simulink model "HQEV_MiL_20160830_integrate"  (Simulink 8.3)
settings: Solver=FixedStepDiscrete  StartTime=0.0  StopTime=inf  FixedStep=0.01  RelTol=1e-3
PostLoadFcn:
  | , if any(exist('dsrtsu_mdlpostloadfcn', 'file') == [2, 3, 6]), try dsrtsu_mdlpostloadfcn('Execute', bdroot); catch fprintf('Error in PostLoadFcn (dsrtsu_mdlpostloadfcn) for model "%s":\n %s\n', bdroot, lasterr); end, end,
values from neighbouring files (symbols this model uses):
  Bat_C_Ah = 36    [parameter_V1.mat]
  Bat_ocv_xIndex = [5 10 20 30 40 50 60 70 80 90 95]    [parameter_V1.mat]
  Bat_ocv_z = [329 332 340 345 347 351 358 372 377 386 391]    [parameter_V1.mat]
  Bat_R_ohm_z = [4.41 3.46 1.57 1.07 0.76 0.63 0.55 0.44 0.41 0.4 0.4 3.14 ... (66 elements, 11x6)]    [parameter_V1.mat]
  Bat_SOC_Init = 90    [parameter_V1.mat]
  Env_hum_pct_Ambient = 30    [parameter_V1.mat]
  Env_Slope_deg = 0    [parameter_V1.mat]
  Env_Temp_degC_Ambient = 25    [parameter_V1.mat]
  Env_v_kmph_HWind = 0    [parameter_V1.mat]
  Reducer_F_i = 7.23    [parameter_V1.mat]
  Reducer_R_i = 7.23    [parameter_V1.mat]
  Veh =     [parameter_V1.mat]
  Veh_A_m2_Fr = 2.246    [parameter_V1.mat]
  Veh_F_Brake =     [parameter_V1.mat]
  Veh_fac_AirDrag = 0.326    [parameter_V1.mat]
  Veh_fac_WhDragFrict_0 = 0.011    [parameter_V1.mat]
  Veh_g_mps2_C = 9.81    [parameter_V1.mat]
  Veh_GainBrake =     [parameter_V1.mat]
  Veh_h_m_COGHigh = 0.5    [parameter_V1.mat]
  Veh_J_kgm2_Wh = 1.3635    [parameter_V1.mat]
  Veh_L_m_AxlBas = 2.63    [parameter_V1.mat]
  Veh_M_kg = 1427    [parameter_V1.mat]
  Veh_mu_Brake = 0.4    [parameter_V1.mat]
  Veh_mu_Tyre =     [parameter_V1.mat]
  Veh_num_FrictPair = 8    [parameter_V1.mat]
  Veh_pct_Brk = 70    [parameter_V1.mat]
  Veh_r_dyn =     [parameter_V1.mat]
  Veh_r_m_BrkDisk = 0.136    [parameter_V1.mat]
  Veh_rho_kgpm3_Air = 1.2258    [parameter_V1.mat]
undefined symbols (not defined in the file or in its folder): DiscIntNeverNeededParam, p_bool_False_M, p_bool_True_M
libraries: BaseOperationLib_Browser x38, simulink x9, DTQC_lib x1, ERR_lib x1, MQM_lib x1, PTCL_lib x1, PUD_lib x1, TQD_lib x1, TQR_lib x1, VMM_lib x1, ACCA_lib x1, BBCA_lib x1
(part 1 of 15)
settings Model: DSRTSU_INTERNAL_RTI_VER=380  DSRTSU_INTERNAL_RTI_TYPE=rti1401  RTICANMMDATA=struct('GeneralSetupData',struct('modelroot','G:\2015\A0EV\MIL_Model_1118\200_Model\230_Integration','generalsettings',struct('filesettings',struct('destfolder',struct('Name','RTICANMM_FILES','Check',1),'buildfolder',struct('Name','.','Check',1),'AbsDestfolder',struct('Name','G:\2015\A0EV\MIL_Model_1118\200_Model\230_Integration\RTICANMM_FILES'),'AbsBuildfolder',struct('Name','G:\2015\A0EV\MIL_Model_1118\200_Model\230_Integration'))),'options',struct('addpaths',1,'rmpaths',1,'addtrcexclusion',logical(1),'cannavigator',struct('checkmonitoring',0,'serviceno','31','hostservicedefheader',struct('name','x','path','x')),'show_usrtrc',0,'use_usrtrc',0),'advanced',struct('options',[1 1 1 1 1 1 1 1 1 1 1 1 1 1 1 1 1 1 1 1 1 1 1 1 1 1 1 1 1 1 1 1 1 1 1 1 1 1 1 1 1 1 1 1 1 1 1 1 1 1 1 1 1 1 1 1 1 1 1 1 1 1 1 1 1 1 1 1 1 1 1 1 1 1 1 1 1 1 1 1 1 1 1 1 1 1 1 1 1 1 1 1 1 1 1 1 1 1 1 1]),'MPSetup',{{}},'modelname','A0EV_HuanJing_1214','block','A0EV_HuanJing_1214'))  Creator=wuaibin  LastModifiedBy=yangfuchun
settings DataIOCC: SaveFormat=StructureWithTime
settings OptimizationCC: BlockReduction=off  ExpressionDepthLimit=2147483647
settings DebuggingCC: FcnCallInpInsideContextMsg=UseLocalSettings
settings HardwareCC: ProdIntDivRoundTo=Zero  ProdEndianess=BigEndian  ProdHWDeviceType=Generic->Custom  TargetIntDivRoundTo=Zero  TargetEndianess=BigEndian  TargetHWDeviceType=Generic->Custom
settings RTWCC: GenerateMakefile=off  TemplateMakefile=grt_msvc.tmf  Description="Visual C/C++ Project Makefile only for the \"grt\" target"  ProcessScript=grt_make_rtw_hook

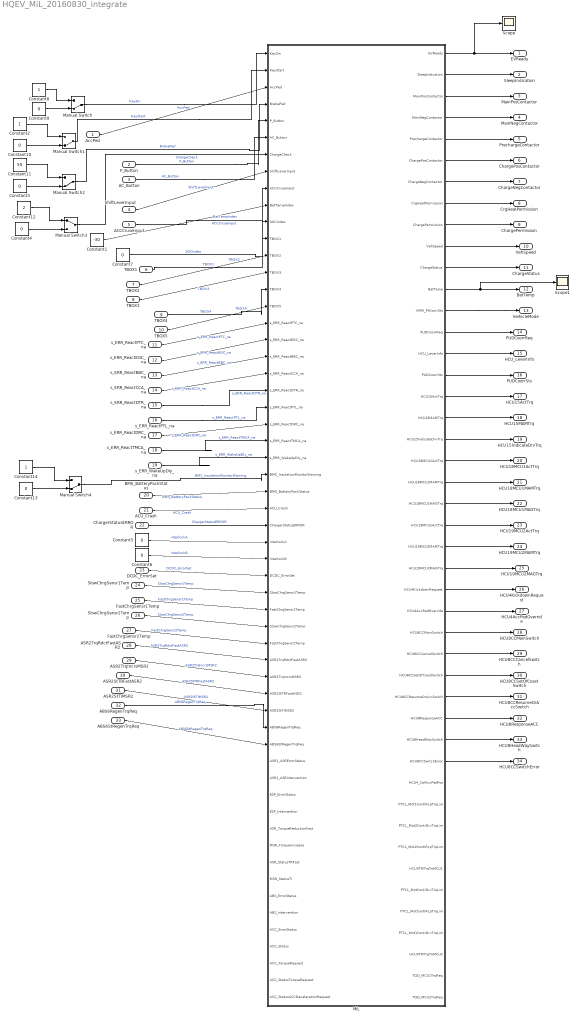
== system HQEV_MiL_20160830_integrate ==
  AccPed : Inport
  P_Button : Inport  Port=2
  AC_Button : Inport  Port=3
  ShiftLeverInput : Inport  Port=4
  ACCCruseInput : Inport  Port=5
  TBOX1 : Inport  Port=6
  TBOX2 : Inport  Port=7
  TBOX3 : Inport  Port=8
  TBOX4 : Inport  Port=9
  TBOX5 : Inport  Port=10
  s_ERR_ReactPTC_na : Inport  Port=11
  s_ERR_ReactEGC_na : Inport  Port=12
  s_ERR_ReactBBC_na : Inport  Port=13
  s_ERR_ReactCCA_na : Inport  Port=14
  s_ERR_ReactDTR_na : Inport  Port=15
  s_ERR_ReactPTL_na : Inport  Port=16
  s_ERR_ReactDRC_na : Inport  Port=17
  s_ERR_ReactTMCA_na : Inport  Port=18
  s_ERR_WakeUpDly_na : Inport  Port=19
  BMS_BatteryPackStatus : Inport  Port=20
  ACU_Crash : Inport  Port=21
  ChargerStatusERROR : Inport  Port=22
  DCDC_ErrorSet : Inport  Port=23
  SlowChrgSensr1Temp : Inport  Port=24
  FastChrgSensr1Temp : Inport  Port=25
  SlowChrgSensr2Temp : Inport  Port=26
  FastChrgSensr2Temp : Inport  Port=27
  ASR2TrqRdctFastASR2 : Inport  Port=28
  ASR2TrqIncrsMSR2 : Inport  Port=29
  ASR2StTRFastASR2 : Inport  Port=30
  ASR2StTIMSR2 : Inport  Port=31
  ABS6RegenTrqReq : Inport  Port=32
  ABS6StRegenTrqReq : Inport  Port=33
  Constant1 : Constant  Value=-30
  Constant{3..7,9..10,13} (8 alike) : Constant  Value=0
  Constant11 : Constant  Value=50
  Constant12 : Constant  Value=2
  Constant14 : Constant
  Constant2 : Constant
  Constant8 : Constant
  Manual Switch{,1..2,4} (4 alike) : ManualSwitch  CurrentSetting=0
  Manual Switch3 : ManualSwitch
  MiL : Subsystem
  Scope : Scope
      settings: YMin=1.9  YMax=2.1
  Scope1 : Scope
      settings: YMin=1.9  YMax=2.1
  EVReady : Outport
  SleepIndication : Outport  Port=2
  MainPosContactor : Outport  Port=3
  MainNegContactor : Outport  Port=4
  PrechargeContactor : Outport  Port=5
  ChargePosContactor : Outport  Port=6
  ChargeNegContactor : Outport  Port=7
  CrgHeatPermission : Outport  Port=8
  ChargePermission : Outport  Port=9
  VehSpeed : Outport  Port=10
  ChargeStatus : Outport  Port=11
  BatTemp : Outport  Port=12
  VeihicleMode : Outport  Port=13
  PUDCoorrReq : Outport  Port=14
  HCU_LeverInfo : Outport  Port=15
  PUDCoorrSts : Outport  Port=16
  HCU15ActTrq : Outport  Port=17
  HCU15MAMTrq : Outport  Port=18
  HCU15IndicateDrvTrq : Outport  Port=19
  HCU18MCU1ActTrq : Outport  Port=20
  HCU18MCU1MAMTrq : Outport  Port=21
  HCU18MCU1MAGTrq : Outport  Port=22
  HCU19MCU2ActTrq : Outport  Port=23
  HCU19MCU2MAMTrq : Outport  Port=24
  HCU19MCU2MAGTrq : Outport  Port=25
  HCU4KickdownRequest : Outport  Port=26
  HCU4AccPedOverride : Outport  Port=27
  HCU8CCMainSwitch : Outport  Port=28
  HCU8CCCancelSwitch : Outport  Port=29
  HCU8CCSetOfCoastSwitch : Outport  Port=30
  HCU8CCResumeOrAccSwitch : Outport  Port=31
  HCU8ResponseACC : Outport  Port=32
  HCU8HeadWaySwitch : Outport  Port=33
  HCU8CCSwitchError : Outport  Port=34
  wires:
  MiL/9(ChargePermission) -> ChargePermission/1
  MiL/4(MainNegContactor) -> MainNegContactor/1
  MiL/1(EVReady) -> Scope/1, EVReady/1
  MiL/3(MainPosContactor) -> MainPosContactor/1
  MiL/7(ChargeNegContactor) -> ChargeNegContactor/1
  MiL/2(SleepIndication) -> SleepIndication/1
  MiL/5(PrechargeContactor) -> PrechargeContactor/1
  MiL/8(CrgHeatPermission) -> CrgHeatPermission/1
  MiL/6(ChargePosContactor) -> ChargePosContactor/1
  MiL/10(VehSpeed) -> VehSpeed/1
  MiL/11(ChargeStatus) -> ChargeStatus/1
  MiL/12(BatTemp) -> Scope1/1, BatTemp/1
  ShiftLeverInput/1 -> MiL/8(ShiftLeverInput)  "ShiftLeverInput"
  P_Button/1 -> MiL/5(P_Button)  "P_Button"
  Constant1/1 -> MiL/10(BatTempIndex)  "BatTempIndex"
  TBOX4/1 -> MiL/15(TBOX4)  "TBOX4"
  TBOX3/1 -> MiL/14(TBOX3)  "TBOX3"
  TBOX5/1 -> MiL/16(TBOX5)  "TBOX5"
  s_ERR_ReactTMCA_na/1 -> MiL/24(s_ERR_ReactTMCA_na)  "s_ERR_ReactTMCA_na"
  s_ERR_ReactPTC_na/1 -> MiL/17(s_ERR_ReactPTC_na)  "s_ERR_ReactPTC_na"
  s_ERR_ReactPTL_na/1 -> MiL/22(s_ERR_ReactPTL_na)  "s_ERR_ReactPTL_na"
  s_ERR_ReactDRC_na/1 -> MiL/23(s_ERR_ReactDRC_na)  "s_ERR_ReactDRC_na"
  s_ERR_ReactCCA_na/1 -> MiL/20(s_ERR_ReactCCA_na)  "s_ERR_ReactCCA_na"
  s_ERR_ReactBBC_na/1 -> MiL/19(s_ERR_ReactBBC_na)  "s_ERR_ReactBBC_na"
  s_ERR_ReactEGC_na/1 -> MiL/18(s_ERR_ReactEGC_na)  "s_ERR_ReactEGC_na"
  s_ERR_ReactDTR_na/1 -> MiL/21(s_ERR_ReactDTR_na)  "s_ERR_ReactDTR_na"
  s_ERR_WakeUpDly_na/1 -> MiL/25(s_ERR_WakeUpDly_na)  "s_ERR_WakeUpDly_na"
  ACCCruseInput/1 -> MiL/9(ACCCruseInput)  "ACCCruseInput"
  TBOX1/1 -> MiL/12(TBOX1)  "TBOX1"
  Constant7/1 -> MiL/11(SOCIndex)  "SOCIndex"
  TBOX2/1 -> MiL/13(TBOX2)  "TBOX2"
  AC_Button/1 -> MiL/6(AC_Button)  "AC_Button"
  Manual Switch1/1 -> MiL/2(KeyStart)  "KeyStart"
  Manual Switch/1 -> MiL/1(KeyOn)  "KeyOn"
  AccPed/1 -> MiL/3(AccPed)  "AccPed"
  Manual Switch2/1 -> MiL/4(BrakePed)  "BrakePed"
  Manual Switch3/1 -> MiL/7(ChargeCheck)  "ChargeCheck"
  Manual Switch4/1 -> MiL/26(BMS_InsulationMonitorWarning)  "BMS_InsulationMonitorWarning"
  BMS_BatteryPackStatus/1 -> MiL/27(BMS_BatteryPackStatus)  "BMS_BatteryPackStatus"
  ACU_Crash/1 -> MiL/28(ACU_Crash)  "ACU_Crash"
  ChargerStatusERROR/1 -> MiL/29(ChargerStatusERROR)  "ChargerStatusERROR"
  Constant5/1 -> MiL/30(interlockA)  "interlockA"
  Constant6/1 -> MiL/31(interlockB)  "interlockB"
  DCDC_ErrorSet/1 -> MiL/32(DCDC_ErrorSet)  "DCDC_ErrorSet"
  SlowChrgSensr1Temp/1 -> MiL/33(SlowChrgSensr1Temp)  "SlowChrgSensr1Temp"
  FastChrgSensr1Temp/1 -> MiL/34(FastChrgSensr1Temp)  "FastChrgSensr1Temp"
  FastChrgSensr2Temp/1 -> MiL/36(FastChrgSensr2Temp)  "FastChrgSensr2Temp"
  SlowChrgSensr2Temp/1 -> MiL/35(SlowChrgSensr2Temp)  "SlowChrgSensr2Temp"
  ASR2StTIMSR2/1 -> MiL/40(ASR2StTIMSR2)  "ASR2StTIMSR2"
  ABS6StRegenTrqReq/1 -> MiL/42(ABS6StRegenTrqReq)  "ABS6StRegenTrqReq"
  ABS6RegenTrqReq/1 -> MiL/41(ABS6RegenTrqReq)  "ABS6RegenTrqReq"
  ASR2TrqIncrsMSR2/1 -> MiL/38(ASR2TrqIncrsMSR2)  "ASR2TrqIncrsMSR2"
  ASR2TrqRdctFastASR2/1 -> MiL/37(ASR2TrqRdctFastASR2)  "ASR2TrqRdctFastASR2"
  ASR2StTRFastASR2/1 -> MiL/39(ASR2StTRFastASR2)  "ASR2StTRFastASR2"
  MiL/13(VMM_PtCoorrSts) -> VeihicleMode/1
  MiL/14(PUDCoorrReq) -> PUDCoorrReq/1
  MiL/15(HCU_LeverInfo) -> HCU_LeverInfo/1
  MiL/16(PUDCoorrSts) -> PUDCoorrSts/1
  MiL/26(HCU4KickdownRequest) -> HCU4KickdownRequest/1
  MiL/17(HCU15ActTrq) -> HCU15ActTrq/1
  MiL/19(HCU15IndicateDrvTrq) -> HCU15IndicateDrvTrq/1
  MiL/18(HCU15MAMTrq) -> HCU15MAMTrq/1
  MiL/20(HCU18MCU1ActTrq) -> HCU18MCU1ActTrq/1
  MiL/21(HCU18MCU1MAMTrq) -> HCU18MCU1MAMTrq/1
  MiL/22(HCU18MCU1MAGTrq) -> HCU18MCU1MAGTrq/1
  MiL/23(HCU19MCU2ActTrq) -> HCU19MCU2ActTrq/1
  MiL/24(HCU19MCU2MAMTrq) -> HCU19MCU2MAMTrq/1
  MiL/25(HCU19MCU2MAGTrq) -> HCU19MCU2MAGTrq/1
  MiL/27(HCU4AccPedOverride) -> HCU4AccPedOverride/1
  MiL/28(HCU8CCMainSwitch) -> HCU8CCMainSwitch/1
  MiL/29(HCU8CCCancelSwitch) -> HCU8CCCancelSwitch/1
  MiL/30(HCU8CCSetOfCoastSwitch) -> HCU8CCSetOfCoastSwitch/1
  MiL/31(HCU8CCResumeOrAccSwitch) -> HCU8CCResumeOrAccSwitch/1
  MiL/32(HCU8ResponseACC) -> HCU8ResponseACC/1
  MiL/33(HCU8HeadWaySwitch) -> HCU8HeadWaySwitch/1
  MiL/34(HCU8CCSwitchError) -> HCU8CCSwitchError/1
  Constant8/1 -> Manual Switch/1
  Constant9/1 -> Manual Switch/2
  Constant2/1 -> Manual Switch1/1
  Constant10/1 -> Manual Switch1/2
  Constant11/1 -> Manual Switch2/1
  Constant3/1 -> Manual Switch2/2
  Constant12/1 -> Manual Switch3/1
  Constant4/1 -> Manual Switch3/2
  Constant14/1 -> Manual Switch4/1
  Constant13/1 -> Manual Switch4/2

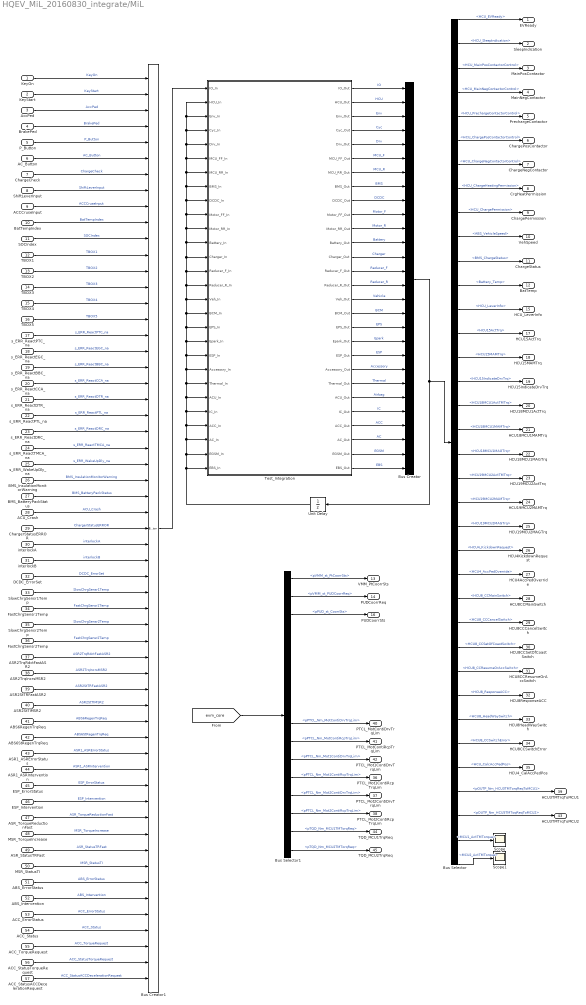
== system HQEV_MiL_20160830_integrate/MiL ==
  KeyOn : Inport
  KeyStart : Inport  Port=2
  AccPed : Inport  Port=3
  BrakePed : Inport  Port=4
  P_Button : Inport  Port=5
  AC_Button : Inport  Port=6
  ChargeCheck : Inport  Port=7
  ShiftLeverInput : Inport  Port=8
  ACCCruseInput : Inport  Port=9
  BatTempIndex : Inport  Port=10
  SOCIndex : Inport  Port=11
  TBOX1 : Inport  Port=12
  TBOX2 : Inport  Port=13
  TBOX3 : Inport  Port=14
  TBOX4 : Inport  Port=15
  TBOX5 : Inport  Port=16
  s_ERR_ReactPTC_na : Inport  Port=17
  s_ERR_ReactEGC_na : Inport  Port=18
  s_ERR_ReactBBC_na : Inport  Port=19
  s_ERR_ReactCCA_na : Inport  Port=20
  s_ERR_ReactDTR_na : Inport  Port=21
  s_ERR_ReactPTL_na : Inport  Port=22
  s_ERR_ReactDRC_na : Inport  Port=23
  s_ERR_ReactTMCA_na : Inport  Port=24
  s_ERR_WakeUpDly_na : Inport  Port=25
  BMS_InsulationMonitorWarning : Inport  Port=26
  BMS_BatteryPackStatus : Inport  Port=27
  ACU_Crash : Inport  Port=28
  ChargerStatusERROR : Inport  Port=29
  interlockA : Inport  Port=30
  interlockB : Inport  Port=31
  DCDC_ErrorSet : Inport  Port=32
  SlowChrgSensr1Temp : Inport  Port=33
  FastChrgSensr1Temp : Inport  Port=34
  SlowChrgSensr2Temp : Inport  Port=35
  FastChrgSensr2Temp : Inport  Port=36
  ASR2TrqRdctFastASR2 : Inport  Port=37
  ASR2TrqIncrsMSR2 : Inport  Port=38
  ASR2StTRFastASR2 : Inport  Port=39
  ASR2StTIMSR2 : Inport  Port=40
  ABS6RegenTrqReq : Inport  Port=41
  ABS6StRegenTrqReq : Inport  Port=42
  ASR1_ASRErrorStatus : Inport  Port=43
  ASR1_ASRIntervention : Inport  Port=44
  ESP_ErrorStatus : Inport  Port=45
  ESP_Intervention : Inport  Port=46
  ASR_TorqueReductionFast : Inport  Port=47
  MSR_TorqueIncrease : Inport  Port=48
  ASR_StatusTRFast : Inport  Port=49
  MSR_StatusTI : Inport  Port=50
  ABS_ErrorStatus : Inport  Port=51
  ABS_Intervention : Inport  Port=52
  ACC_ErrorStatus : Inport  Port=53
  ACC_Status : Inport  Port=54
  ACC_TorqueRequest : Inport  Port=55
  ACC_StatusTorqueRequest : Inport  Port=56
  ACC_StatusACCDecelerationRequest : Inport  Port=57
  Bus Creator : BusCreator  Inputs=28
  Bus Creator1 : BusCreator  Inputs=57
  Bus Selector : BusSelector  OutputSignals=HCU.HCU_EVReady,HCU.HCU_SleepIndication,HCU.HCU_MainPosContactorControl,HCU.HCU_MainNegContactorControl,HCU.HCU_PrechargeContactorControl,HCU.HCU_ChargePosContactorControl,HCU.HCU_ChargeNegContactorControl,HCU.HCU_ChargeHeatingPermission,HCU.HCU_ChargePermission,ESP.ABS.ABS_VehicleSpeed,BMS.BMS_ChargeStatus,Thermal.Battery_Temp,HCU.HCU_LeverInfo,HCU.PT_HCU_15.HCU15ActTrq,HCU.PT_HCU_15.HCU15MAMTrq,HCU.PT_HCU_15.HCU15IndicateDrvTrq,HCU.PT_HCU_18.HCU18MCU1ActTMTrq,HCU.PT_HCU_18.HCU18MCU1MAMTrq,HCU.PT_HCU_18.HCU18MCU1MAGTrq,HCU.PT_HCU_19.HCU19MCU2ActTMTrq,HCU.PT_HCU_19.HCU19MCU2MAMTrq,HCU.PT_HCU_19.HCU19MCU2MAGTrq,HCU.PT_HCU_4.HCU4_KickdownRequest,HCU.PT_HCU_4.HCU4_AccPedOverride,HCU.PT_HCU_8.HCU8_CCMainSwitch,HCU.PT_HCU_8.HCU8_CCCancelSwitch,HCU.PT_HCU_8.HCU8_CCSetOfCoastSwitch,HCU.PT_HCU_8.HCU8_CCResumeOrAccSwitch,HCU.PT_HCU_8.HCU8_ResponseACC,HCU.PT_HCU_8.HCU8_HeadWaySwitch,HCU.PT_HCU_8.HCU8_CCSwitchError,HCU.PT_HCU_4.HCU_CalcAccPedPos,HCU.HCU_OUT.HCU_EVCAN.EV_HCU_3.pOUTP_Nm_HCU3TMTorqReqToMCU1,HCU.HCU_OUT.HCU_EVCAN.EV_HCU_5.pOUTP_Nm_HCU5TMToqReqToMCU2,MCU_F.MCU1_ActTMTorque,MCU_R.MCU2_ActTMTorque
  Bus Selector1 : BusSelector  OutputSignals=Bus_VMM.pVMM_st_PtCoorrSts,Bus_VMM.pVMM_st_PUDCoorrReq,Bus_PUD.pPUD_st_CoorrSts,Bus_PUD.pPUD_st_AcChrgModeSt,Bus_PUD.pPUD_st_DcChrgModeSt,Bus_PUD.pPUD_st_AcHeatModeSt,Bus_PUD.pPUD_st_DcHeatModeSt,Bus_PUD.pPUD_st_HVOnModeSt,Bus_PTCL.pPTCL_Nm_MotContiDrvTrqLim,Bus_PTCL.pPTCL_Nm_MotContiRcpTrqLim,Bus_PTCL.pPTCL_Nm_Mot1ContiDrvTrqLim,Bus_PTCL.pPTCL_Nm_Mot1ContiRcpTrqLim,Bus_PTCL.pPTCL_Nm_Mot2ContiDrvTrqLim,Bus_PTCL.pPTCL_Nm_Mot2ContiRcpTrqLim,Bus_TQD.pTQD_Nm_MCU1TMTorqReq,Bus_TQD.pTQD_Nm_MCU2TMTorqReq
  Scope : Scope
      settings: SaveName=ScopeData3
  Scope1 : Scope
      settings: SaveName=ScopeData6
  Test_Integration : Subsystem
  Unit Delay : UnitDelay  SampleTime=-1
  EVReady : Outport
  SleepIndication : Outport  Port=2
  MainPosContactor : Outport  Port=3
  MainNegContactor : Outport  Port=4
  PrechargeContactor : Outport  Port=5
  ChargePosContactor : Outport  Port=6
  ChargeNegContactor : Outport  Port=7
  CrgHeatPermission : Outport  Port=8
  ChargePermission : Outport  Port=9
  VehSpeed : Outport  Port=10
  ChargeStatus : Outport  Port=11
  BatTemp : Outport  Port=12
  VMM_PtCoorrSts : Outport  Port=13
  PUDCoorrReq : Outport  Port=14
  HCU_LeverInfo : Outport  Port=15
  PUDCoorrSts : Outport  Port=16
  HCU15ActTrq : Outport  Port=17
  HCU15MAMTrq : Outport  Port=18
  HCU15IndicateDrvTrq : Outport  Port=19
  HCU18MCU1ActTrq : Outport  Port=20
  HCU18MCU1MAMTrq : Outport  Port=21
  HCU18MCU1MAGTrq : Outport  Port=22
  HCU19MCU2ActTrq : Outport  Port=23
  HCU19MCU2MAMTrq : Outport  Port=24
  HCU19MCU2MAGTrq : Outport  Port=25
  HCU4KickdownRequest : Outport  Port=26
  HCU4AccPedOverride : Outport  Port=27
  HCU8CCMainSwitch : Outport  Port=28
  HCU8CCCancelSwitch : Outport  Port=29
  HCU8CCSetOfCoastSwitch : Outport  Port=30
  HCU8CCResumeOrAccSwitch : Outport  Port=31
  HCU8ResponseACC : Outport  Port=32
  HCU8HeadWaySwitch : Outport  Port=33
  HCU8CCSwitchError : Outport  Port=34
  HCU4_CalAccPedPos : Outport  Port=35
  PTCL_Mot1ContiRcpTrqLim : Outport  Port=36
  PTCL_Mot2ContiDrvTrqLim : Outport  Port=37
  PTCL_Mot2ContiRcpTrqLim : Outport  Port=38
  HCU3TMTrqToMCU1 : Outport  Port=39
  PTCL_MotContiDrvTrqLim : Outport  Port=40
  PTCL_MotContiRcpTrqLim : Outport  Port=41
  PTCL_Mot1ContiDrvTrqLim : Outport  Port=42
  HCU3TMTrqToMCU2 : Outport  Port=43
  TQD_MCU1TrqReq : Outport  Port=44
  TQD_MCU2TrqReq : Outport  Port=45
  wires:
  ShiftLeverInput/1 -> Bus Creator1/8  "ShiftLeverInput"
  Test_Integration/1(IO_Out) -> Bus Creator/1  "IO"
  Test_Integration/2(HCU_Out) -> Bus Creator/2  "HCU"
  Test_Integration/3(Env_Out) -> Bus Creator/3  "Env"
  Test_Integration/4(Cyc_Out) -> Bus Creator/4  "Cyc"
  Test_Integration/5(Drv_Out) -> Bus Creator/5  "Drv"
  Test_Integration/6(MCU_FF_Out) -> Bus Creator/6  "MCU_F"
  Test_Integration/7(MCU_RR_Out) -> Bus Creator/7  "MCU_R"
  Test_Integration/8(BMS_Out) -> Bus Creator/8  "BMS"
  Test_Integration/9(DCDC_Out) -> Bus Creator/9  "DCDC"
  Test_Integration/10(Motor_FF_Out) -> Bus Creator/10  "Motor_F"
  Test_Integration/11(Motor_RR_Out) -> Bus Creator/11  "Motor_R"
  Test_Integration/12(Battery_Out) -> Bus Creator/12  "Battery"
  Test_Integration/13(Charger_Out) -> Bus Creator/13  "Charger"
  Test_Integration/14(Reducer_F_Out) -> Bus Creator/14  "Reducer_F"
  Test_Integration/15(Reducer_R_Out) -> Bus Creator/15  "Reducer_R"
  Test_Integration/16(Veh_Out) -> Bus Creator/16  "Vehicle"
  Test_Integration/17(BCM_Out) -> Bus Creator/17  "BCM"
  Test_Integration/18(EPS_Out) -> Bus Creator/18  "EPS"
  Test_Integration/19(Epark_Out) -> Bus Creator/19  "Epark"
  Test_Integration/20(ESP_Out) -> Bus Creator/20  "ESP"
  Test_Integration/21(Accessory_Out) -> Bus Creator/21  "Accessory"
  Test_Integration/22(Thermal_Out) -> Bus Creator/22  "Thermal"
  Test_Integration/23(ACU_Out) -> Bus Creator/23  "Airbag"
  Test_Integration/24(IC_Out) -> Bus Creator/24  "IC"
  Test_Integration/25(ACC_Out) -> Bus Creator/25  "ACC"
  Bus Creator/1 -> Unit Delay/1, Bus Selector/1
  Test_Integration/26(AC_Out) -> Bus Creator/26  "AC"
  Test_Integration/27(EGSM_Out) -> Bus Creator/27  "EGSM"
  Test_Integration/28(EBS_Out) -> Bus Creator/28  "EBS"
  Unit Delay/1 -> Test_Integration/2(HCU_In), Test_Integration/3(Env_In), Test_Integration/4(Cyc_In), Test_Integration/5(Drv_In), Test_Integration/6(MCU_FF_In), Test_Integration/7(MCU_RR_In), Test_Integration/8(BMS_In), Test_Integration/9(DCDC_In), Test_Integration/10(Motor_FF_In), Test_Integration/11(Motor_RR_In), Test_Integration/12(Battery_In), Test_Integration/13(Charger_In), Test_Integration/14(Reducer_F_In), Test_Integration/15(Reducer_R_In), Test_Integration/16(Veh_In), Test_Integration/17(BCM_In), Test_Integration/18(EPS_In), Test_Integration/19(Epark_In), Test_Integration/20(ESP_In), Test_Integration/21(Accesssry_In), Test_Integration/22(Thermal_In), Test_Integration/23(ACU_In), Test_Integration/24(IC_In), Test_Integration/25(ACC_In), Test_Integration/26(AC_In), Test_Integration/27(EGSM_In), Test_Integration/28(EBS_In)
  Bus Creator1/1 -> Test_Integration/1(IO_In)
  P_Button/1 -> Bus Creator1/5  "P_Button"
  BatTempIndex/1 -> Bus Creator1/10  "BatTempIndex"
  TBOX4/1 -> Bus Creator1/15  "TBOX4"
  TBOX3/1 -> Bus Creator1/14  "TBOX3"
  TBOX5/1 -> Bus Creator1/16  "TBOX5"
  s_ERR_ReactTMCA_na/1 -> Bus Creator1/24  "s_ERR_ReactTMCA_na"
  s_ERR_ReactPTC_na/1 -> Bus Creator1/17  "s_ERR_ReactPTC_na"
  s_ERR_ReactPTL_na/1 -> Bus Creator1/22  "s_ERR_ReactPTL_na"
  s_ERR_ReactDRC_na/1 -> Bus Creator1/23  "s_ERR_ReactDRC_na"
  s_ERR_ReactCCA_na/1 -> Bus Creator1/20  "s_ERR_ReactCCA_na"
  s_ERR_ReactBBC_na/1 -> Bus Creator1/19  "s_ERR_ReactBBC_na"
  s_ERR_ReactEGC_na/1 -> Bus Creator1/18  "s_ERR_ReactEGC_na"
  s_ERR_ReactDTR_na/1 -> Bus Creator1/21  "s_ERR_ReactDTR_na"
  s_ERR_WakeUpDly_na/1 -> Bus Creator1/25  "s_ERR_WakeUpDly_na"
  ACCCruseInput/1 -> Bus Creator1/9  "ACCCruseInput"
  TBOX1/1 -> Bus Creator1/12  "TBOX1"
  SOCIndex/1 -> Bus Creator1/11  "SOCIndex"
  TBOX2/1 -> Bus Creator1/13  "TBOX2"
  AC_Button/1 -> Bus Creator1/6  "AC_Button"
  KeyStart/1 -> Bus Creator1/2  "KeyStart"
  KeyOn/1 -> Bus Creator1/1  "KeyOn"
  AccPed/1 -> Bus Creator1/3  "AccPed"
  BrakePed/1 -> Bus Creator1/4  "BrakePed"
  ChargeCheck/1 -> Bus Creator1/7  "ChargeCheck"
  Bus Selector/9 -> ChargePermission/1  "<HCU_ChargePermission>"
  Bus Selector/8 -> CrgHeatPermission/1  "<HCU_ChargeHeatingPermission>"
  Bus Selector/7 -> ChargeNegContactor/1  "<HCU_ChargeNegContactorControl>"
  Bus Selector/5 -> PrechargeContactor/1  "<HCU_PrechargeContactorControl>"
  Bus Selector/3 -> MainPosContactor/1  "<HCU_MainPosContactorControl>"
  Bus Selector/1 -> EVReady/1  "<HCU_EVReady>"
  Bus Selector/4 -> MainNegContactor/1  "<HCU_MainNegContactorControl>"
  Bus Selector/2 -> SleepIndication/1  "<HCU_SleepIndication>"
  Bus Selector/6 -> ChargePosContactor/1  "<HCU_ChargePosContactorControl>"
  Bus Selector/10 -> VehSpeed/1  "<ABS_VehicleSpeed>"
  Bus Selector/11 -> ChargeStatus/1  "<BMS_ChargeStatus>"
  Bus Selector/12 -> BatTemp/1  "<Battery_Temp>"
  [evm_core] -> Bus Selector1/1
  Bus Selector1/1 -> VMM_PtCoorrSts/1  "<pVMM_st_PtCoorrSts>"
  Bus Selector1/2 -> PUDCoorrReq/1  "<pVMM_st_PUDCoorrReq>"
  Bus Selector/13 -> HCU_LeverInfo/1  "<HCU_LeverInfo>"
  BMS_InsulationMonitorWarning/1 -> Bus Creator1/26  "BMS_InsulationMonitorWarning"
  BMS_BatteryPackStatus/1 -> Bus Creator1/27  "BMS_BatteryPackStatus"
  ACU_Crash/1 -> Bus Creator1/28  "ACU_Crash"
  ChargerStatusERROR/1 -> Bus Creator1/29  "ChargerStatusERROR"
  interlockA/1 -> Bus Creator1/30  "interlockA"
  interlockB/1 -> Bus Creator1/31  "interlockB"
  DCDC_ErrorSet/1 -> Bus Creator1/32  "DCDC_ErrorSet"
  SlowChrgSensr1Temp/1 -> Bus Creator1/33  "SlowChrgSensr1Temp"
  FastChrgSensr1Temp/1 -> Bus Creator1/34  "FastChrgSensr1Temp"
  FastChrgSensr2Temp/1 -> Bus Creator1/36  "FastChrgSensr2Temp"
  SlowChrgSensr2Temp/1 -> Bus Creator1/35  "SlowChrgSensr2Temp"
  Bus Selector1/3 -> PUDCoorrSts/1  "<pPUD_st_CoorrSts>"
  ASR2StTIMSR2/1 -> Bus Creator1/40  "ASR2StTIMSR2"
  ABS6StRegenTrqReq/1 -> Bus Creator1/42  "ABS6StRegenTrqReq"
  ABS6RegenTrqReq/1 -> Bus Creator1/41  "ABS6RegenTrqReq"
  ASR2TrqIncrsMSR2/1 -> Bus Creator1/38  "ASR2TrqIncrsMSR2"
  ASR2TrqRdctFastASR2/1 -> Bus Creator1/37  "ASR2TrqRdctFastASR2"
  ASR2StTRFastASR2/1 -> Bus Creator1/39  "ASR2StTRFastASR2"
  Bus Selector/20 -> HCU19MCU2ActTrq/1  "<HCU19MCU2ActTMTrq>"
  Bus Selector/15 -> HCU15MAMTrq/1  "<HCU15MAMTrq>"
  Bus Selector/26 -> HCU8CCCancelSwitch/1  "<HCU8_CCCancelSwitch>"
  Bus Selector/23 -> HCU4KickdownRequest/1  "<HCU4_KickdownRequest>"
  Bus Selector/14 -> HCU15ActTrq/1  "<HCU15ActTrq>"
  Bus Selector/24 -> HCU4AccPedOverride/1  "<HCU4_AccPedOverride>"
  Bus Selector/18 -> HCU18MCU1MAMTrq/1  "<HCU18MCU1MAMTrq>"
  Bus Selector/16 -> HCU15IndicateDrvTrq/1  "<HCU15IndicateDrvTrq>"
  Bus Selector/22 -> HCU19MCU2MAGTrq/1  "<HCU19MCU2MAGTrq>"
  Bus Selector/19 -> HCU18MCU1MAGTrq/1  "<HCU18MCU1MAGTrq>"
  Bus Selector/25 -> HCU8CCMainSwitch/1  "<HCU8_CCMainSwitch>"
  Bus Selector/21 -> HCU19MCU2MAMTrq/1  "<HCU19MCU2MAMTrq>"
  Bus Selector/17 -> HCU18MCU1ActTrq/1  "<HCU18MCU1ActTMTrq>"
  Bus Selector/28 -> HCU8CCResumeOrAccSwitch/1  "<HCU8_CCResumeOrAccSwitch>"
  Bus Selector/27 -> HCU8CCSetOfCoastSwitch/1  "<HCU8_CCSetOfCoastSwitch>"
  Bus Selector/29 -> HCU8ResponseACC/1  "<HCU8_ResponseACC>"
  Bus Selector/30 -> HCU8HeadWaySwitch/1  "<HCU8_HeadWaySwitch>"
  Bus Selector/31 -> HCU8CCSwitchError/1  "<HCU8_CCSwitchError>"
  ASR1_ASRErrorStatus/1 -> Bus Creator1/43  "ASR1_ASRErrorStatus"
  ASR1_ASRIntervention/1 -> Bus Creator1/44  "ASR1_ASRIntervention"
  ESP_ErrorStatus/1 -> Bus Creator1/45  "ESP_ErrorStatus"
  ESP_Intervention/1 -> Bus Creator1/46  "ESP_Intervention"
  ASR_TorqueReductionFast/1 -> Bus Creator1/47  "ASR_TorqueReductionFast"
  MSR_TorqueIncrease/1 -> Bus Creator1/48  "MSR_TorqueIncrease"
  ASR_StatusTRFast/1 -> Bus Creator1/49  "ASR_StatusTRFast"
  MSR_StatusTI/1 -> Bus Creator1/50  "MSR_StatusTI"
  ABS_ErrorStatus/1 -> Bus Creator1/51  "ABS_ErrorStatus"
  ABS_Intervention/1 -> Bus Creator1/52  "ABS_Intervention"
  ACC_ErrorStatus/1 -> Bus Creator1/53  "ACC_ErrorStatus"
  ACC_Status/1 -> Bus Creator1/54  "ACC_Status"
  ACC_TorqueRequest/1 -> Bus Creator1/55  "ACC_TorqueRequest"
  ACC_StatusTorqueRequest/1 -> Bus Creator1/56  "ACC_StatusTorqueRequest"
  ACC_StatusACCDecelerationRequest/1 -> Bus Creator1/57  "ACC_StatusACCDecelerationRequest"
  Bus Selector/32 -> HCU4_CalAccPedPos/1  "<HCU_CalcAccPedPos>"
  Bus Selector1/14 -> PTCL_Mot2ContiRcpTrqLim/1  "<pPTCL_Nm_Mot2ContiRcpTrqLim>"
  Bus Selector1/13 -> PTCL_Mot2ContiDrvTrqLim/1  "<pPTCL_Nm_Mot2ContiDrvTrqLim>"
  Bus Selector1/12 -> PTCL_Mot1ContiRcpTrqLim/1  "<pPTCL_Nm_Mot1ContiRcpTrqLim>"
  Bus Selector1/11 -> PTCL_Mot1ContiDrvTrqLim/1  "<pPTCL_Nm_Mot1ContiDrvTrqLim>"
  Bus Selector1/10 -> PTCL_MotContiRcpTrqLim/1  "<pPTCL_Nm_MotContiRcpTrqLim>"
  Bus Selector1/9 -> PTCL_MotContiDrvTrqLim/1  "<pPTCL_Nm_MotContiDrvTrqLim>"
  Bus Selector/33 -> HCU3TMTrqToMCU1/1  "<pOUTP_Nm_HCU3TMTorqReqToMCU1>"
  Bus Selector/34 -> HCU3TMTrqToMCU2/1  "<pOUTP_Nm_HCU5TMToqReqToMCU2>"
  Bus Selector1/15 -> TQD_MCU1TrqReq/1  "<pTQD_Nm_MCU1TMTorqReq>"
  Bus Selector1/16 -> TQD_MCU2TrqReq/1  "<pTQD_Nm_MCU2TMTorqReq>"
  Bus Selector/35 -> Scope/1  "<MCU1_ActTMTorque>"
  Bus Selector/36 -> Scope1/1  "<MCU2_ActTMTorque>"

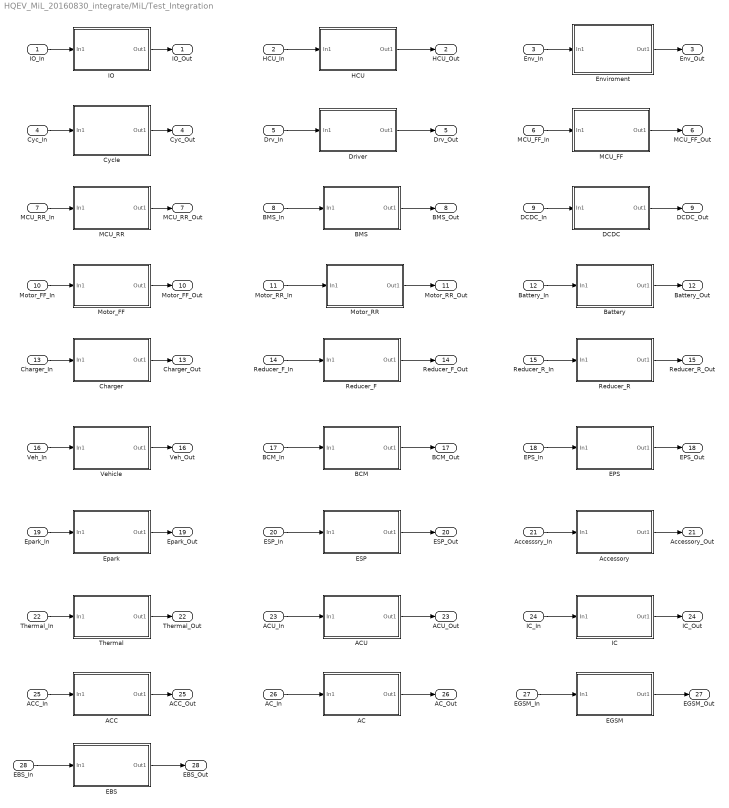
== system HQEV_MiL_20160830_integrate/MiL/Test_Integration ==
  IO_In : Inport
  HCU_In : Inport  Port=2
  Env_In : Inport  Port=3
  Cyc_In : Inport  Port=4
  Drv_In : Inport  Port=5
  MCU_FF_In : Inport  Port=6
  MCU_RR_In : Inport  Port=7
  BMS_In : Inport  Port=8
  DCDC_In : Inport  Port=9
  Motor_FF_In : Inport  Port=10
  Motor_RR_In : Inport  Port=11
  Battery_In : Inport  Port=12
  Charger_In : Inport  Port=13
  Reducer_F_In : Inport  Port=14
  Reducer_R_In : Inport  Port=15
  Veh_In : Inport  Port=16
  BCM_In : Inport  Port=17
  EPS_In : Inport  Port=18
  Epark_In : Inport  Port=19
  ESP_In : Inport  Port=20
  Accesssry_In : Inport  Port=21
  Thermal_In : Inport  Port=22
  ACU_In : Inport  Port=23
  IC_In : Inport  Port=24
  ACC_In : Inport  Port=25
  AC_In : Inport  Port=26
  EGSM_In : Inport  Port=27
  EBS_In : Inport  Port=28
  AC : Subsystem
  ACC : Subsystem
  ACU : Subsystem
  Accessory : Subsystem
  BCM : Subsystem
  BMS : Subsystem
  Battery : Subsystem
  Charger : Subsystem
  Cycle : Subsystem
  DCDC : Subsystem
  Driver : Subsystem
  EBS : Subsystem
  EGSM : Subsystem
  EPS : Subsystem
  ESP : Subsystem
  Enviroment : Subsystem
  Epark : Subsystem
  HCU : Subsystem
  IC : Subsystem
  IO : Subsystem
  MCU_FF : Subsystem
  MCU_RR : Subsystem
  Motor_FF : Subsystem
  Motor_RR : Subsystem
  Reducer_F : Subsystem
  Reducer_R : Subsystem
  Thermal : Subsystem
  Vehicle : Subsystem
  IO_Out : Outport
  HCU_Out : Outport  Port=2
  Env_Out : Outport  Port=3
  Cyc_Out : Outport  Port=4
  Drv_Out : Outport  Port=5
  MCU_FF_Out : Outport  Port=6
  MCU_RR_Out : Outport  Port=7
  BMS_Out : Outport  Port=8
  DCDC_Out : Outport  Port=9
  Motor_FF_Out : Outport  Port=10
  Motor_RR_Out : Outport  Port=11
  Battery_Out : Outport  Port=12
  Charger_Out : Outport  Port=13
  Reducer_F_Out : Outport  Port=14
  Reducer_R_Out : Outport  Port=15
  Veh_Out : Outport  Port=16
  BCM_Out : Outport  Port=17
  EPS_Out : Outport  Port=18
  Epark_Out : Outport  Port=19
  ESP_Out : Outport  Port=20
  Accessory_Out : Outport  Port=21
  Thermal_Out : Outport  Port=22
  ACU_Out : Outport  Port=23
  IC_Out : Outport  Port=24
  ACC_Out : Outport  Port=25
  AC_Out : Outport  Port=26
  EGSM_Out : Outport  Port=27
  EBS_Out : Outport  Port=28
  wires:
  HCU_In/1 -> HCU/1(In1)
  HCU/1(Out1) -> HCU_Out/1
  Env_In/1 -> Enviroment/1(In1)
  Enviroment/1(Out1) -> Env_Out/1
  Cyc_In/1 -> Cycle/1(In1)
  Cycle/1(Out1) -> Cyc_Out/1
  Drv_In/1 -> Driver/1(In1)
  Driver/1(Out1) -> Drv_Out/1
  MCU_FF_In/1 -> MCU_FF/1(In1)
  MCU_FF/1(Out1) -> MCU_FF_Out/1
  MCU_RR_In/1 -> MCU_RR/1(In1)
  MCU_RR/1(Out1) -> MCU_RR_Out/1
  BMS_In/1 -> BMS/1(In1)
  BMS/1(Out1) -> BMS_Out/1
  DCDC_In/1 -> DCDC/1(In1)
  DCDC/1(Out1) -> DCDC_Out/1
  Charger_In/1 -> Charger/1(In1)
  Charger/1(Out1) -> Charger_Out/1
  Veh_In/1 -> Vehicle/1(In1)
  Vehicle/1(Out1) -> Veh_Out/1
  Reducer_R/1(Out1) -> Reducer_R_Out/1
  Reducer_R_In/1 -> Reducer_R/1(In1)
  Reducer_F/1(Out1) -> Reducer_F_Out/1
  Reducer_F_In/1 -> Reducer_F/1(In1)
  Battery_In/1 -> Battery/1(In1)
  Motor_RR/1(Out1) -> Motor_RR_Out/1
  Motor_RR_In/1 -> Motor_RR/1(In1)
  Motor_FF/1(Out1) -> Motor_FF_Out/1
  Motor_FF_In/1 -> Motor_FF/1(In1)
  Battery/1(Out1) -> Battery_Out/1
  IO_In/1 -> IO/1(In1)
  IO/1(Out1) -> IO_Out/1
  Thermal_In/1 -> Thermal/1(In1)
  Thermal/1(Out1) -> Thermal_Out/1
  BCM_In/1 -> BCM/1(In1)
  BCM/1(Out1) -> BCM_Out/1
  EPS_In/1 -> EPS/1(In1)
  EPS/1(Out1) -> EPS_Out/1
  Epark_In/1 -> Epark/1(In1)
  Epark/1(Out1) -> Epark_Out/1
  ESP_In/1 -> ESP/1(In1)
  ESP/1(Out1) -> ESP_Out/1
  Accesssry_In/1 -> Accessory/1(In1)
  Accessory/1(Out1) -> Accessory_Out/1
  ACU_In/1 -> ACU/1(In1)
  ACU/1(Out1) -> ACU_Out/1
  IC_In/1 -> IC/1(In1)
  IC/1(Out1) -> IC_Out/1
  ACC_In/1 -> ACC/1(In1)
  ACC/1(Out1) -> ACC_Out/1
  AC_In/1 -> AC/1(In1)
  AC/1(Out1) -> AC_Out/1
  EGSM_In/1 -> EGSM/1(In1)
  EGSM/1(Out1) -> EGSM_Out/1
  EBS_In/1 -> EBS/1(In1)
  EBS/1(Out1) -> EBS_Out/1

== system HQEV_MiL_20160830_integrate/MiL/Test_Integration/AC ==
  In1 : Inport
  AirConditioning : Subsystem
  Unit Delay : UnitDelay  SampleTime=-1
  Out1 : Outport
  wires:
  Unit Delay/1 -> Out1/1
  AirConditioning/1(AC) -> Unit Delay/1
  In1/1 -> AirConditioning/1(In1)

== system HQEV_MiL_20160830_integrate/MiL/Test_Integration/ACC ==
  In1 : Inport
  ACC : Subsystem
  Unit Delay : UnitDelay  SampleTime=-1
  Out1 : Outport
  wires:
  ACC/1(ACC) -> Unit Delay/1
  In1/1 -> ACC/1(In1)
  Unit Delay/1 -> Out1/1

== system HQEV_MiL_20160830_integrate/MiL/Test_Integration/ACU ==
  In1 : Inport
  ACU : Subsystem
  Bus Creator : BusCreator
  Unit Delay : UnitDelay  SampleTime=-1
  Out1 : Outport
  wires:
  In1/1 -> ACU/1(In1)
  ACU/1(Checksum_ACU_1) -> Bus Creator/1  "Checksum_ACU_1"
  ACU/2(ACU_Crash) -> Bus Creator/2  "ACU_Crash"
  ACU/3(LiveCounter_ACU_1) -> Bus Creator/3  "LiveCounter_ACU_1"
  ACU/4(ACU_ErrorStatus) -> Bus Creator/4  "ACU_ErrorStatus"
  Bus Creator/1 -> Unit Delay/1
  Unit Delay/1 -> Out1/1

== system HQEV_MiL_20160830_integrate/MiL/Test_Integration/Accessory ==
  In1 : Inport
  Accessory : Subsystem
  Out1 : Outport
  wires:
  In1/1 -> Accessory/1(In1)
  Accessory/1(Out1) -> Out1/1

== system HQEV_MiL_20160830_integrate/MiL/Test_Integration/BCM ==
  In1 : Inport
  BCM : Subsystem
  Unit Delay : UnitDelay  SampleTime=-1
  Out1 : Outport
  wires:
  In1/1 -> BCM/1(In1)
  BCM/1(BCM) -> Unit Delay/1
  Unit Delay/1 -> Out1/1

== system HQEV_MiL_20160830_integrate/MiL/Test_Integration/BMS ==
  In1 : Inport
  BMS : Subsystem
  Unit Delay : UnitDelay  SampleTime=-1
  Out1 : Outport
  wires:
  In1/1 -> BMS/1(In1)
  BMS/1(Out1) -> Unit Delay/1
  Unit Delay/1 -> Out1/1

== system HQEV_MiL_20160830_integrate/MiL/Test_Integration/Battery ==
  In1 : Inport
  Battery : Subsystem
  Out1 : Outport
  wires:
  In1/1 -> Battery/1(In)
  Battery/1(Out) -> Out1/1

== system HQEV_MiL_20160830_integrate/MiL/Test_Integration/Charger ==
  In1 : Inport
  Charger : Subsystem
  Unit Delay : UnitDelay  SampleTime=-1
  Out1 : Outport
  wires:
  In1/1 -> Charger/1(In1)
  Charger/1(Out) -> Unit Delay/1
  Unit Delay/1 -> Out1/1

== system HQEV_MiL_20160830_integrate/MiL/Test_Integration/Cycle ==
  In1 : Inport
  Cycle : Subsystem
  Out1 : Outport
  wires:
  In1/1 -> Cycle/1(In1)
  Cycle/1(Out1) -> Out1/1

== system HQEV_MiL_20160830_integrate/MiL/Test_Integration/DCDC ==
  In1 : Inport
  DCDC : Subsystem
  Unit Delay : UnitDelay  SampleTime=-1
  Out1 : Outport
  wires:
  In1/1 -> DCDC/1(In1)
  DCDC/1(Out1) -> Unit Delay/1
  Unit Delay/1 -> Out1/1

== system HQEV_MiL_20160830_integrate/MiL/Test_Integration/Driver ==
  In1 : Inport
  Bus Selector : BusSelector  OutputSignals=Vehicle.v_Veh,Cyc.v_set,IO
  Driver : Subsystem
  Out1 : Outport
  wires:
  Driver/1(Out1) -> Out1/1
  In1/1 -> Bus Selector/1
  Bus Selector/1 -> Driver/1(v_Veh)  "<v_Veh>"
  Bus Selector/2 -> Driver/2(Cycle_v_set)  "<v_set>"
  Bus Selector/3 -> Driver/3(IO_IN)  "<IO>"

== system HQEV_MiL_20160830_integrate/MiL/Test_Integration/EBS ==
  In1 : Inport
  Bus Creator : BusCreator  Inputs=7
  EBS : Subsystem
  Unit Delay : UnitDelay  SampleTime=-1
  Out1 : Outport
  wires:
  In1/1 -> EBS/1(In1)
  EBS/1(SOC) -> Bus Creator/1  "SOC"
  EBS/2(T_BATT) -> Bus Creator/2  "T_BATT"
  EBS/3(Status_Temp) -> Bus Creator/3  "Status_Temp"
  EBS/4(ERROR_Calib) -> Bus Creator/4  "ERROR_Calib"
  EBS/5(Resp_Error) -> Bus Creator/5  "Resp_Error"
  EBS/6(FLAG_INCONSISTENCY) -> Bus Creator/6  "FLAG_INCONSISTENCY"
  EBS/7(SOC_STATE) -> Bus Creator/7  "SOC_STATE"
  Bus Creator/1 -> Unit Delay/1
  Unit Delay/1 -> Out1/1

== system HQEV_MiL_20160830_integrate/MiL/Test_Integration/EGSM ==
  In1 : Inport
  Bus Creator : BusCreator  Inputs=12
  EGSM : Subsystem
  Unit Delay : UnitDelay  SampleTime=-1
  Out1 : Outport
  wires:
  EGSM/1(Checksum_EGSM_1) -> Bus Creator/1  "Checksum_EGSM_1"
  EGSM/2(EGSM_ParkButton) -> Bus Creator/2  "EGSM_ParkButton"
  EGSM/3(EGSM_SecurityButton) -> Bus Creator/3  "EGSM_SecurityButton"
  EGSM/4(EGSM_KnobPosition) -> Bus Creator/4  "EGSM_KnobPosition"
  EGSM/5(EGSMErrorStatus) -> Bus Creator/5  "EGSMErrorStatus"
  EGSM/6(EGSM_ECOSButton) -> Bus Creator/6  "EGSM_ECOSButton"
  EGSM/7(LiveCounter_EGSM_1) -> Bus Creator/7  "LiveCounter_EGSM_1"
  EGSM/8(PowerSupplyStatus) -> Bus Creator/8  "PowerSupplyStatus"
  EGSM/9(EGSM_CANError) -> Bus Creator/9  "EGSM_CANError"
  EGSM/10(EGSM_LINError) -> Bus Creator/10  "EGSM_LINError"
  EGSM/11(EGSM_HallSensorError) -> Bus Creator/11  "EGSM_HallSensorError"
  EGSM/12(EGSM_InternalError) -> Bus Creator/12  "EGSM_InternalError"
  Bus Creator/1 -> Unit Delay/1
  Unit Delay/1 -> Out1/1
  In1/1 -> EGSM/1(In1)

== system HQEV_MiL_20160830_integrate/MiL/Test_Integration/EPS ==
  In1 : Inport
  EPS : Subsystem
  Terminator : Terminator
  Out1 : Outport
  wires:
  In1/1 -> Terminator/1
  EPS/1(EPS) -> Out1/1

== system HQEV_MiL_20160830_integrate/MiL/Test_Integration/ESP ==
  In1 : Inport
  Subsystem : Subsystem
  Unit Delay : UnitDelay  SampleTime=-1
  Out1 : Outport
  wires:
  In1/1 -> Subsystem/1(In1)
  Subsystem/1(ESP) -> Unit Delay/1
  Unit Delay/1 -> Out1/1

== system HQEV_MiL_20160830_integrate/MiL/Test_Integration/Enviroment ==
  In1 : Inport
  Bus Creator : BusCreator
  Environment : Subsystem
  Terminator : Terminator
  Unit Delay : UnitDelay  SampleTime=-1
  Out1 : Outport
  wires:
  In1/1 -> Terminator/1
  Bus Creator/1 -> Unit Delay/1
  Environment/1(Slope_deg) -> Bus Creator/1  "Slope"
  Environment/2(v_Hwind_mps) -> Bus Creator/2  "v_Hwind"
  Environment/3(Temp_Amb_degC) -> Bus Creator/3  "Temp_Amb"
  Environment/4(Theta_Air_pct) -> Bus Creator/4  "Theta_Air"
  Unit Delay/1 -> Out1/1

== system HQEV_MiL_20160830_integrate/MiL/Test_Integration/Epark ==
  In1 : Inport
  Subsystem : Subsystem
  Out1 : Outport
  wires:
  In1/1 -> Subsystem/1(In1)
  Subsystem/1(out) -> Out1/1

== system HQEV_MiL_20160830_integrate/MiL/Test_Integration/HCU ==
  In1 : Inport
  Bus Creator : BusCreator  Inputs=43
  HCU : Subsystem
  Unit Delay : UnitDelay  SampleTime=-1
  Out1 : Outport
  wires:
  Unit Delay/1 -> Out1/1
  In1/1 -> HCU/1(In1)
  HCU/1(ACU_Crash) -> Bus Creator/1  "ACU_Crash"
  HCU/2(HCU_DCDCOutputVoltageRequest) -> Bus Creator/2  "HCU_DCDCOutputVoltageRequest"
  HCU/3(HCU_DCDCEnable) -> Bus Creator/3  "HCU_DCDCEnable"
  HCU/4(HCU_MainPosContactorControl) -> Bus Creator/4  "HCU_MainPosContactorControl"
  HCU/5(HCU_MainNegContactorControl) -> Bus Creator/5  "HCU_MainNegContactorControl"
  HCU/6(HCU_PrechargeContactorControl) -> Bus Creator/6  "HCU_PrechargeContactorControl"
  HCU/7(HCU_ChargePosContactorControl) -> Bus Creator/7  "HCU_ChargePosContactorControl"
  Bus Creator/1 -> Unit Delay/1
  HCU/8(HCU_ChargeNegContactorControl) -> Bus Creator/8  "HCU_ChargeNegContactorControl"
  HCU/9(HCU_SleepIndication) -> Bus Creator/9  "HCU_SleepIndication"
  HCU/10(HCU_ChargeHeatingPermission) -> Bus Creator/10  "HCU_ChargeHeatingPermission"
  HCU/11(HCU_ChargeConnectStatus) -> Bus Creator/11  "HCU_ChargeConnectStatus"
  HCU/12(HCU_ChargePermission) -> Bus Creator/12  "HCU_ChargePermission"
  HCU/13(HCU_VehicleOperatingMode) -> Bus Creator/13  "HCU_VehicleOperatingMode"
  HCU/14(HCU_TMTorqueRequestToMCU1) -> Bus Creator/14  "HCU_TMTorqueRequestToMCU1"
  HCU/15(HCU_StatusTMRequestToMCU1) -> Bus Creator/15  "HCU_StatusTMRequestToMCU1"
  HCU/16(HCU_StopRequestToMCU1) -> Bus Creator/16  "HCU_StopRequestToMCU1"
  HCU/17(HCU_RapidDischargeCmdToMCU1) -> Bus Creator/17  "HCU_RapidDischargeCmdToMCU1"
  HCU/18(HCU_AntiJerkDisableCmdToMCU1) -> Bus Creator/18  "HCU_AntiJerkDisableCmdToMCU1"
  HCU/19(HCU_TMTorqueRequestToMCU2) -> Bus Creator/19  "HCU_TMTorqueRequestToMCU2"
  HCU/20(HCU_StatusTMRequestToMCU2) -> Bus Creator/20  "HCU_StatusTMRequestToMCU2"
  HCU/21(HCU_StopRequestToMCU2) -> Bus Creator/21  "HCU_StopRequestToMCU2"
  HCU/22(HCU_RapidDischargeCmdToMCU2) -> Bus Creator/22  "HCU_RapidDischargeCmdToMCU2"
  HCU/23(HCU_AntiJerkDisableCmdToMCU2) -> Bus Creator/23  "HCU_AntiJerkDisableCmdToMCU2"
  HCU/24(HCU_VehicleDeiceHeatPermit) -> Bus Creator/24  "HCU_VehicleDeiceHeatPermit"
  HCU/25(HCU_BatteryPackCoolRequest) -> Bus Creator/25  "HCU_BatteryPackCoolRequest"
  HCU/26(HCU_IGOFFRequest) -> Bus Creator/26  "HCU_IGOFFRequest"
  HCU/27(HCU_BatterySOCWarning) -> Bus Creator/27  "HCU_BatterySOCWarning"
  HCU/28(HCU_EVReady) -> Bus Creator/28  "HCU_EVReady"
  HCU/29(HCU_Status) -> Bus Creator/29  "HCU_Status"
  HCU/30(HCU_ParkRequest) -> Bus Creator/30  "HCU_ParkRequest"
  HCU/31(PTC_PWM_pct) -> Bus Creator/31  "PTC_PWM_pct"
  HCU/32(LowSpdFanCmd_na) -> Bus Creator/32  "LowSpdFanCmd_na"
  HCU/33(HighSpdFanCmd_na) -> Bus Creator/33  "HighSpdFanCmd_na"
  HCU/34(EM1PumpCmd_pct) -> Bus Creator/34  "EM1PumpCmd_pct"
  HCU/35(EM2PumpCmd_pct) -> Bus Creator/35  "EM2PumpCmd_pct"
  HCU/36(BatPumpCmd_pct) -> Bus Creator/36  "BatPumpCmd_pct"
  HCU/37(HCU_LeverInfo) -> Bus Creator/37  "HCU_LeverInfo"
  HCU/38(PT_HCU_15) -> Bus Creator/38  "PT_HCU_15"
  HCU/39(PT_HCU_18) -> Bus Creator/39  "PT_HCU_18"
  HCU/40(PT_HCU_19) -> Bus Creator/40  "PT_HCU_19"
  HCU/41(PT_HCU_4) -> Bus Creator/41  "PT_HCU_4"
  HCU/42(PT_HCU_8) -> Bus Creator/42  "PT_HCU_8"
  HCU/43(HCU_Out) -> Bus Creator/43  "HCU_OUT"

== system HQEV_MiL_20160830_integrate/MiL/Test_Integration/IC ==
  In1 : Inport
  IC : Subsystem
  Unit Delay : UnitDelay  SampleTime=-1
  Out1 : Outport
  wires:
  In1/1 -> IC/1(In1)
  IC/1(IC) -> Unit Delay/1
  Unit Delay/1 -> Out1/1

== system HQEV_MiL_20160830_integrate/MiL/Test_Integration/IO ==
  In1 : Inport
  Out1 : Outport
  wires:
  In1/1 -> Out1/1

== system HQEV_MiL_20160830_integrate/MiL/Test_Integration/MCU_FF ==
  In1 : Inport
  MCU : Subsystem
  Out1 : Outport
  wires:
  In1/1 -> MCU/1(In1)
  MCU/1(Out1) -> Out1/1

== system HQEV_MiL_20160830_integrate/MiL/Test_Integration/MCU_RR ==
  In1 : Inport
  MCU : Subsystem
  Out1 : Outport
  wires:
  In1/1 -> MCU/1(In1)
  MCU/1(Out1) -> Out1/1

== system HQEV_MiL_20160830_integrate/MiL/Test_Integration/Motor_FF ==
  In1 : Inport
  Motor : Subsystem
  Out1 : Outport
  wires:
  In1/1 -> Motor/1(In1)
  Motor/1(Out1) -> Out1/1

== system HQEV_MiL_20160830_integrate/MiL/Test_Integration/Motor_RR ==
  In1 : Inport
  Motor : Subsystem
  Out1 : Outport
  wires:
  In1/1 -> Motor/1(In1)
  Motor/1(Out1) -> Out1/1

== system HQEV_MiL_20160830_integrate/MiL/Test_Integration/Reducer_F ==
  In1 : Inport
  FinalDrive : Subsystem
  Out1 : Outport
  wires:
  In1/1 -> FinalDrive/1(In1)
  FinalDrive/1(Out) -> Out1/1

== system HQEV_MiL_20160830_integrate/MiL/Test_Integration/Reducer_R ==
  In1 : Inport
  FinalDrive : Subsystem
  Out1 : Outport
  wires:
  In1/1 -> FinalDrive/1(In1)
  FinalDrive/1(Out) -> Out1/1

== system HQEV_MiL_20160830_integrate/MiL/Test_Integration/Thermal ==
  In1 : Inport
  Thermal : Subsystem
  Unit Delay : UnitDelay  SampleTime=-1
  Out1 : Outport
  wires:
  In1/1 -> Thermal/1(In1)
  Thermal/1(Out1) -> Unit Delay/1
  Unit Delay/1 -> Out1/1

== system HQEV_MiL_20160830_integrate/MiL/Test_Integration/Vehicle ==
  In1 : Inport
  Vehicle : Subsystem
  Out1 : Outport
  wires:
  In1/1 -> Vehicle/1(In1)
  Vehicle/1(Out2) -> Out1/1

== system HQEV_MiL_20160830_integrate/MiL/Test_Integration/AC/AirConditioning ==
  In1 : Inport
  ACIndication : Subsystem
  AC_CompressorOnRequest : Subsystem
  AC_FanRequest : Subsystem
  AC_PTCStatus : Subsystem
  AC_PowerConsumptionH : Subsystem
  AC_PowerConsumptionL : Subsystem
  AC_ShutdownEnableH : Subsystem
  AC_Status : Subsystem
  AC_shutdownEnableL : Subsystem
  BLWLevelIndication : Subsystem
  Bus Creator2 : BusCreator  Inputs=13
  Checksum_AC_1 : Subsystem
  LiveCounter_AC_1 : Subsystem
  OutsideTemperatureIndication : Subsystem
  Terminator : Terminator
  AC : Outport
  wires:
  In1/1 -> Terminator/1
  Checksum_AC_1/1(out) -> Bus Creator2/1  "Checksum_AC_1"
  LiveCounter_AC_1/1(out) -> Bus Creator2/2  "LiveCounter_AC_1"
  AC_CompressorOnRequest/1(out) -> Bus Creator2/3  "AC_CompressorOnRequest"
  AC_Status/1(out) -> Bus Creator2/4  "AC_Status"
  AC_PowerConsumptionL/1(out) -> Bus Creator2/5  "AC_PowerConsumptionL"
  AC_ShutdownEnableH/1(out) -> Bus Creator2/6  "AC_ShutdownEnableH"
  AC_shutdownEnableL/1(out) -> Bus Creator2/7  "AC_shutdownEnableL"
  AC_PTCStatus/1(out) -> Bus Creator2/9  "AC_PTCStatus"
  AC_FanRequest/1(out) -> Bus Creator2/8  "AC_FanRequest"
  AC_PowerConsumptionH/1(out) -> Bus Creator2/10  "AC_PowerConsumptionH"
  ACIndication/1(out) -> Bus Creator2/11  "ACIndication"
  BLWLevelIndication/1(out) -> Bus Creator2/12  "AC_BLWLevelIndication"
  OutsideTemperatureIndication/1(out) -> Bus Creator2/13  "AC_OutsideTemperatureIndication"
  Bus Creator2/1 -> AC/1

== system HQEV_MiL_20160830_integrate/MiL/Test_Integration/ACC/ACC ==
  In1 : Inport
  Bus Creator : BusCreator  Inputs=6
  Ground : Ground
  Output : Subsystem
  ACC : Outport
  wires:
  Bus Creator/1 -> ACC/1
  In1/1 -> Output/17(IO_Input)
  Ground/1 -> Output/4(AccelerationPedalPosition), Output/5(CalculatedAccelerationPedalPosition), Output/6(KickdownRequest), Output/7(BrakeSwitch), Output/8(AccelerationPedalOverride), Output/9(CCMainSwitch), Output/10(CCCancelSwitch), Output/11(CCSetOrCoastSwitch), Output/12(CCResumeOrAccelerateSwitch), Output/13(HCUResponseACC), Output/15(CCSwitchError), Output/16(LeverInfo), Output/14(HeadwaySwitch), Output/3(HCUStatus), Output/2(HCU_MaxAvaiblleMotoringTorque), Output/1(HCU_ActualMotoringTorque)
  Output/4(ACC_StatusTorqueRequest) -> Bus Creator/4  "ACC_StatusTorqueRequest"
  Output/5(ACC_DecelerationRequest) -> Bus Creator/5  "ACC_DecelerationRequest"
  Output/1(ACC_ErrorStatus) -> Bus Creator/1  "ACC_ErrorStatus"
  Output/2(ACC_Status) -> Bus Creator/2  "ACC_Status"
  Output/6(ACC_StatusACCDecelerationRequest) -> Bus Creator/6  "ACC_StatusACCDecelerationRequest"
  Output/3(ACC_TorqueRequest) -> Bus Creator/3  "ACC_TorqueRequest"

== system HQEV_MiL_20160830_integrate/MiL/Test_Integration/ACU/ACU ==
  In1 : Inport
  Bus Selector : BusSelector  OutputSignals=IO.ACU_Crash
  Constant : Constant  Value=0
  Checksum_ACU_1 : Outport
  ACU_Crash : Outport  Port=2
  LiveCounter_ACU_1 : Outport  Port=3
  ACU_ErrorStatus : Outport  Port=4
  wires:
  Constant/1 -> Checksum_ACU_1/1, ACU_ErrorStatus/1, LiveCounter_ACU_1/1
  In1/1 -> Bus Selector/1
  Bus Selector/1 -> ACU_Crash/1  "<ACU_Crash>"

== system HQEV_MiL_20160830_integrate/MiL/Test_Integration/Accessory/Accessory ==
  In1 : Inport
  Bus Creator : BusCreator  Inputs=1
  Subsystem : Subsystem
  Out1 : Outport
  wires:
  Bus Creator/1 -> Out1/1
  In1/1 -> Subsystem/1(In1)
  Subsystem/1(vacuum degree) -> Bus Creator/1  "vacuum degree"

== system HQEV_MiL_20160830_integrate/MiL/Test_Integration/BCM/BCM ==
  In1 : Inport
  Bus Creator : BusCreator  Inputs=7
  Check : Subsystem
  BCM : Outport
  wires:
  In1/1 -> Check/1(In1)
  Check/1(BCM_HighBeamCmd) -> Bus Creator/1  "BCM_HighBeamCmd"
  Check/2(DriverDoorSt) -> Bus Creator/2  "DriverDoorSt"
  Check/3(WiperStatus) -> Bus Creator/3  "WiperStatus"
  Check/4(Checksum_PSC) -> Bus Creator/4  "Checksum_PSC"
  Check/5(DataBytes) -> Bus Creator/5  "DataBytes"
  Check/6(LiveCounter_PSC) -> Bus Creator/6  "LiveCounter_PSC"
  Check/7(MessageType) -> Bus Creator/7  "MessageType"
  Bus Creator/1 -> BCM/1

== system HQEV_MiL_20160830_integrate/MiL/Test_Integration/BMS/BMS ==
  In1 : Inport
  BMS : Subsystem
  Bus Creator1 : BusCreator  Inputs=2
  Signal : Subsystem
  Out1 : Outport
  wires:
  In1/1 -> Bus Creator1/1, BMS/1(In1)
  Bus Creator1/1 -> Signal/1(In1)
  BMS/1(Out) -> Bus Creator1/2  "BMS"
  Signal/1(Out1) -> Out1/1

== system HQEV_MiL_20160830_integrate/MiL/Test_Integration/Battery/Battery ==
  In : Inport
  Battery : Subsystem
  Bus Creator : BusCreator  Inputs=6
  Bus Selector : BusSelector  OutputSignals=Motor_F.EM1_pwr_elec,Motor_R.EM2_pwr_elec,DCDC.DCDC_Input_Powr,AC.AC_PowerConsumptionH,Thermal.Battery_Temp,IO.SOCIndex,Charger.Charger_OutputVoltage,Charger.Charger_OutputCurrent,HCU.HCU_ChargePermission
  Out : Outport
  wires:
  Battery/1(Battery_Voltage) -> Bus Creator/1  "Battery_Voltage"
  Battery/2(Battery_Current) -> Bus Creator/2  "Battery_Current"
  Bus Creator/1 -> Out/1
  Battery/3(SOC) -> Bus Creator/3  "SOC"
  Battery/4(SOH) -> Bus Creator/4  "SOH"
  Battery/5(Battery_Temperature) -> Bus Creator/5  "Battery_Temp"
  Battery/6(Battery_Power_loss) -> Bus Creator/6  "Battery_Power_loss"
  In/1 -> Bus Selector/1
  Bus Selector/1 -> Battery/1(EM1_pwr_elec)  "<EM1_pwr_elec>"
  Bus Selector/2 -> Battery/2(EM2_pwr_elec)  "<EM2_pwr_elec>"
  Bus Selector/3 -> Battery/3(DCDC_pwr_in)  "<DCDC_Input_Powr>"
  Bus Selector/4 -> Battery/4(AC_pwr_elec)  "<AC_PowerConsumptionH>"
  Bus Selector/5 -> Battery/5(Battery_Temp)  "<Battery_Temp>"
  Bus Selector/6 -> Battery/6(SOCIndex)  "<SOCIndex>"
  Bus Selector/7 -> Battery/7(Charger_OutputVoltage)  "<Charger_OutputVoltage>"
  Bus Selector/8 -> Battery/8(Charger_OutputCurrent)  "<Charger_OutputCurrent>"
  Bus Selector/9 -> Battery/9(HCU_ChargerPermission)  "<HCU_ChargePermission>"

== system HQEV_MiL_20160830_integrate/MiL/Test_Integration/Charger/Charger ==
  In1 : Inport
  Charger : Subsystem
  Signal : Subsystem
  Out : Outport
  wires:
  In1/1 -> Charger/1(In)
  Charger/1(Out) -> Signal/1(In)
  Signal/1(out) -> Out/1

== system HQEV_MiL_20160830_integrate/MiL/Test_Integration/Cycle/Cycle ==
  In1 : Inport
  Bus Creator : BusCreator  Inputs=1
  Cycle : Subsystem
  Out1 : Outport
  wires:
  In1/1 -> Cycle/1(In)
  Cycle/1(v_set [km/h]) -> Bus Creator/1  "v_set"
  Bus Creator/1 -> Out1/1

== system HQEV_MiL_20160830_integrate/MiL/Test_Integration/DCDC/DCDC ==
  In1 : Inport
  Bus Creator1 : BusCreator  Inputs=2
  DCDC : Subsystem
  Output : Subsystem
  Out1 : Outport
  wires:
  In1/1 -> DCDC/1(In1), Bus Creator1/1
  DCDC/1(DCDC) -> Bus Creator1/2
  Bus Creator1/1 -> Output/1(In1)
  Output/1(Out1) -> Out1/1

== system HQEV_MiL_20160830_integrate/MiL/Test_Integration/Driver/Driver ==
  v_Veh : Inport
  Cycle_v_set : Inport  Port=2
  IO_IN : Inport  Port=3
  Bus Creator : BusCreator  Inputs=3
  Bus Creator1 : BusCreator  Inputs=3
  Bus Creator2 : BusCreator  Inputs=2
  Control_Panel : Subsystem
  Driver_AutoPedal : Subsystem
  Driver_ManualPedal : Subsystem
  Manual Switch : simulink/Signal Routing/Manual Switch  SystemSampleTime=-1  sw=0  action=0  varsize=off
  Out1 : Outport
  wires:
  v_Veh/1 -> Driver_AutoPedal/1(Veh_v)  "v_Veh"
  Cycle_v_set/1 -> Driver_AutoPedal/2(Cycle_v_set)  "v_Set"
  Driver_AutoPedal/1(AccPed_pct) -> Bus Creator/1  "AccPed_pct"
  Driver_AutoPedal/2(BrkPed_pct) -> Bus Creator/2  "BrkPed_pct"
  Driver_AutoPedal/3(Brake_OnOff) -> Bus Creator/3  "Brake_OnOff"
  Driver_ManualPedal/2(BrkPed_pct) -> Bus Creator1/2  "BrkPed_pct"
  Driver_ManualPedal/3(Brake_OnOff) -> Bus Creator1/3  "Brake_OnOff"
  Bus Creator/1 -> Manual Switch/1
  Bus Creator1/1 -> Manual Switch/2
  Control_Panel/1(Out1) -> Bus Creator2/2
  Manual Switch/1 -> Bus Creator2/1
  Bus Creator2/1 -> Out1/1
  IO_IN/1 -> Driver_ManualPedal/1(IO_IN), Control_Panel/1(IO_IN)
  Driver_ManualPedal/1(AccPed_pct) -> Bus Creator1/1  "AccPed_pct"

== system HQEV_MiL_20160830_integrate/MiL/Test_Integration/EBS/EBS ==
  In1 : Inport
  Subsystem : Subsystem
  Subsystem1 : Subsystem
  Subsystem2 : Subsystem
  Subsystem3 : Subsystem
  Subsystem4 : Subsystem
  Subsystem5 : Subsystem
  Subsystem6 : Subsystem
  Subsystem7 : Subsystem
  Terminator : Terminator
  Terminator1 : Terminator
  SOC : Outport
  T_BATT : Outport  Port=2
  Status_Temp : Outport  Port=3
  ERROR_Calib : Outport  Port=4
  Resp_Error : Outport  Port=5
  FLAG_INCONSISTENCY : Outport  Port=6
  SOC_STATE : Outport  Port=7
  wires:
  Subsystem/1(SOC) -> SOC/1
  Subsystem1/1(T_BATT) -> T_BATT/1
  Subsystem2/1(Status_Temp) -> Status_Temp/1
  Subsystem3/1(ERROR_Calib) -> ERROR_Calib/1
  Subsystem4/1(Resp_Error) -> Resp_Error/1
  Subsystem5/1(FLAG_INCONSISTENCY) -> FLAG_INCONSISTENCY/1
  Subsystem6/1(SOC_STATE) -> SOC_STATE/1
  In1/1 -> Terminator/1
  Subsystem7/1(out) -> Terminator1/1
